simulink library "Sensitive_Room_Temperature"  (Simulink 8.2)
settings: Solver=ode45  StartTime=0.0  StopTime=10.0  RelTol=1e-3
settings Model: Creator=lena.frank  LastModifiedBy=drhf

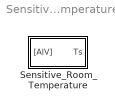
== system Sensitive_Room_Temperature ==
  Sensitive_Room_Temperature : Subsystem  mask(SENSITIVE TEMPERATURE){share_c=47}
      mask prompts: share_c "SHARE of convective sensitivity, [0,100%]:"
      mask help:
      | This block merges the convective and radiative zone node temperature to the SENSITIVE ZONE TEMPERATURE (weighted arithmetic average of both components).
      | [T] = [Tc; Tr]:  temperature vector of node, °C
      | Ts:              sensitive zone temperature, °C
      mask init:
      | blockname = gcb;
      | 
      | if (length(share_c)~=1) error(['PARAMETERS block "' blockname ': "SHARE of ..." must have only 1 entry !']); end;
      | if (share_c<0) | (share_c>100) error(['PARAMETERS block "' blockname '" : "SHARE of ..." must be within [0, 100%] !']); end;
      | share_c = share_c/100;
      mask Help: web(fullfile(path_carnot('help'),'Sensitive_room_temperature.html'),'-helpbrowser')

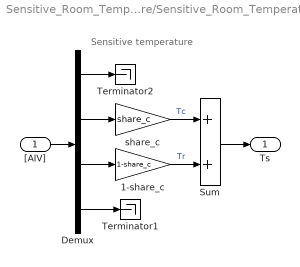
== system Sensitive_Room_Temperature/Sensitive_Room_Temperature ==
  note: Sensitive temperature
  "[AIV]" : Inport
  1-share_c : Gain  Gain=1-share_c  SaturateOnIntegerOverflow=on  OutDataTypeStr=Inherit: Same as input  ParamDataTypeStr=Inherit: Same as input
  Demux : Demux  Outputs=[1 1 1 6]
  Sum : Sum  SaturateOnIntegerOverflow=on  InputSameDT=on  OutDataTypeStr=Inherit: Same as first input
  Terminator1 : Terminator
  Terminator2 : Terminator
  share_c : Gain  Gain=share_c  SaturateOnIntegerOverflow=on  OutDataTypeStr=Inherit: Same as input  ParamDataTypeStr=Inherit: Same as input
  Ts : Outport
  wires:
  Demux/3 -> 1-share_c/1
  Demux/2 -> share_c/1
  "[AIV]"/1 -> Demux/1
  Demux/4 -> Terminator1/1
  share_c/1 -> Sum/1  "Tc"
  1-share_c/1 -> Sum/2  "Tr"
  Sum/1 -> Ts/1
  Demux/1 -> Terminator2/1
